simulink model "fullSystem"  (R2019a)
settings: Solver=ode45  StartTime=0.0  StopTime=70  FixedStep=0.01  RelTol=1e-3
settings Model: Creator=Dario Quintero  LastModifiedBy=dq16394
settings DebuggingCC: PregeneratedLibrarySubsystemCodeDiagnostic=none  ArithmeticOperatorsInVariantConditions=warning

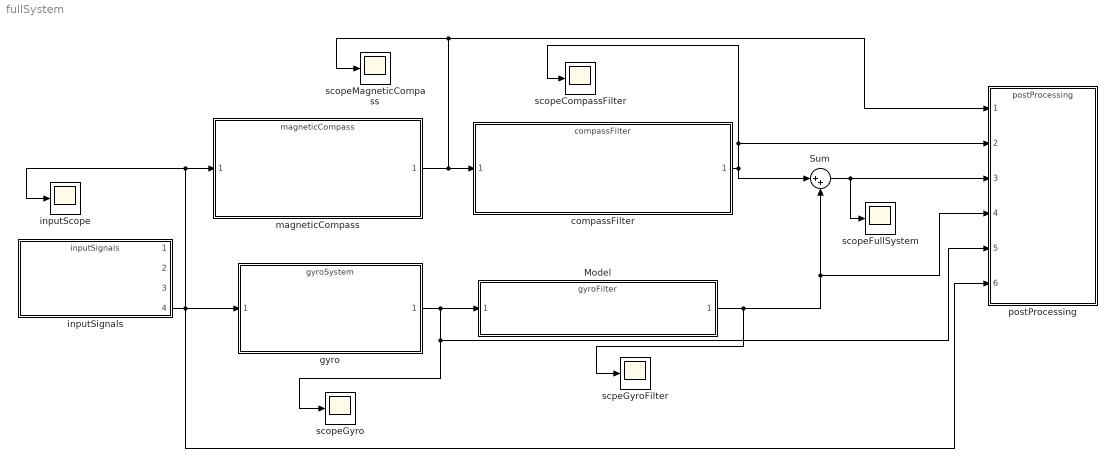
== system fullSystem ==
  Model : ModelReference  ModelNameDialog=gyroFilter.slx  SimulationMode=Normal  ModelReferenceVersion=1.4
  Sum : Sum  Inputs=|++
  compassFilter : ModelReference  ModelNameDialog=compassFilter.slx  SimulationMode=Normal  ModelReferenceVersion=1.4
  gyro : ModelReference  ModelNameDialog=gyroSystem.slx  SimulationMode=Normal  ModelReferenceVersion=1.18
  inputScope : Scope
  inputSignals : ModelReference  ModelNameDialog=inputSignals.slx  SimulationMode=Normal  ModelReferenceVersion=1.25
  magneticCompass : ModelReference  ModelNameDialog=magneticCompass.slx  SimulationMode=Normal  ModelReferenceVersion=1.8
  postProcessing : ModelReference  ModelNameDialog=postProcessing.slx  SimulationMode=Normal  ModelReferenceVersion=1.21
  scopeCompassFilter : Scope
  scopeFullSystem : Scope
  scopeGyro : Scope
  scopeMagneticCompass : Scope
  scpeGyroFilter : Scope
  wires:
  magneticCompass/1 -> scopeMagneticCompass/1, postProcessing/1, compassFilter/1
  gyro/1 -> scopeGyro/1, postProcessing/5, Model/1
  compassFilter/1 -> scopeCompassFilter/1, postProcessing/2, Sum/1
  inputSignals/4 -> inputScope/1, magneticCompass/1, postProcessing/6, gyro/1
  Model/1 -> scpeGyroFilter/1, Sum/2, postProcessing/4
  Sum/1 -> postProcessing/3, scopeFullSystem/1
